simulink model "mw_ssrconverter"  (R2020a)
settings: Solver=VariableStepAuto  StartTime=0.0  StopTime=(8192*2)/256e6  RelTol=1e-3
InitFcn:
  | fs = 256e6;
libraries: hdlsllib x111, simulink x42
(part 1 of 2)
settings Model: EnablePacing=on  PacingRate=0.000001  Creator=david  LastModifiedBy=david
settings OptimizationCC: BlockReduction=off  ConditionallyExecuteInputs=off  DefaultParameterBehavior=Inlined
settings DebuggingCC: AlgebraicLoopMsg=error
settings HardwareCC: ProdBitPerPointer=32  ProdBitPerSizeT=32  ProdBitPerPtrDiffT=32  ProdLargestAtomicFloat=None  ProdIntDivRoundTo=Undefined  ProdEndianess=Unspecified  ProdWordSize=32  ProdHWDeviceType=ASIC/FPGA->ASIC/FPGA  TargetBitPerPointer=64  TargetBitPerSizeT=64  TargetBitPerPtrDiffT=64  TargetLongLongMode=on  TargetIntDivRoundTo=Zero  TargetEndianess=LittleEndian  TargetWordSize=64  TargetHWDeviceType=Custom Processor->MATLAB Host Computer  ProdEqTarget=off

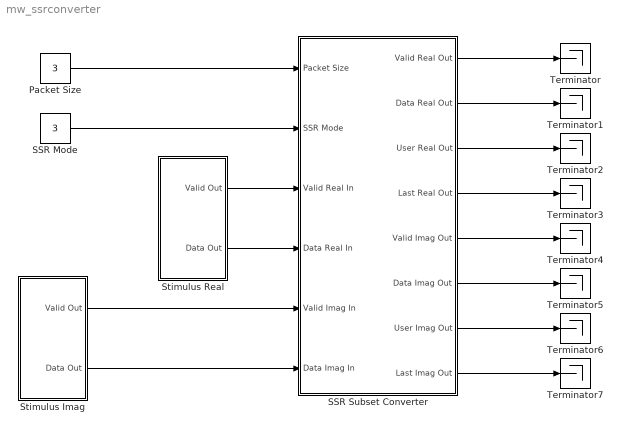
== system mw_ssrconverter ==
  Packet Size : Constant  Value=3  OutDataTypeStr=uint32  SampleTime=-1
  SSR Mode : Constant  Value=3  OutDataTypeStr=uint32  SampleTime=-1
  SSR Subset Converter : Subsystem  TreatAsAtomicUnit=on
  Stimulus Imag : Subsystem
  Stimulus Real : Subsystem
  Terminator{,1..7} (8 alike) : Terminator
  wires:
  Packet Size/1 -> SSR Subset Converter/1(Packet Size)
  SSR Mode/1 -> SSR Subset Converter/2(SSR Mode)
  Stimulus Real/1(Valid Out) -> SSR Subset Converter/3(Valid Real In)
  Stimulus Real/2(Data Out) -> SSR Subset Converter/4(Data Real In)
  SSR Subset Converter/1(Valid Real Out) -> Terminator/1
  SSR Subset Converter/2(Data Real Out) -> Terminator1/1
  SSR Subset Converter/3(User Real Out) -> Terminator2/1
  SSR Subset Converter/4(Last Real Out) -> Terminator3/1
  Stimulus Imag/1(Valid Out) -> SSR Subset Converter/5(Valid Imag In)
  Stimulus Imag/2(Data Out) -> SSR Subset Converter/6(Data Imag In)
  SSR Subset Converter/8(Last Imag Out) -> Terminator7/1
  SSR Subset Converter/7(User Imag Out) -> Terminator6/1
  SSR Subset Converter/6(Data Imag Out) -> Terminator5/1
  SSR Subset Converter/5(Valid Imag Out) -> Terminator4/1

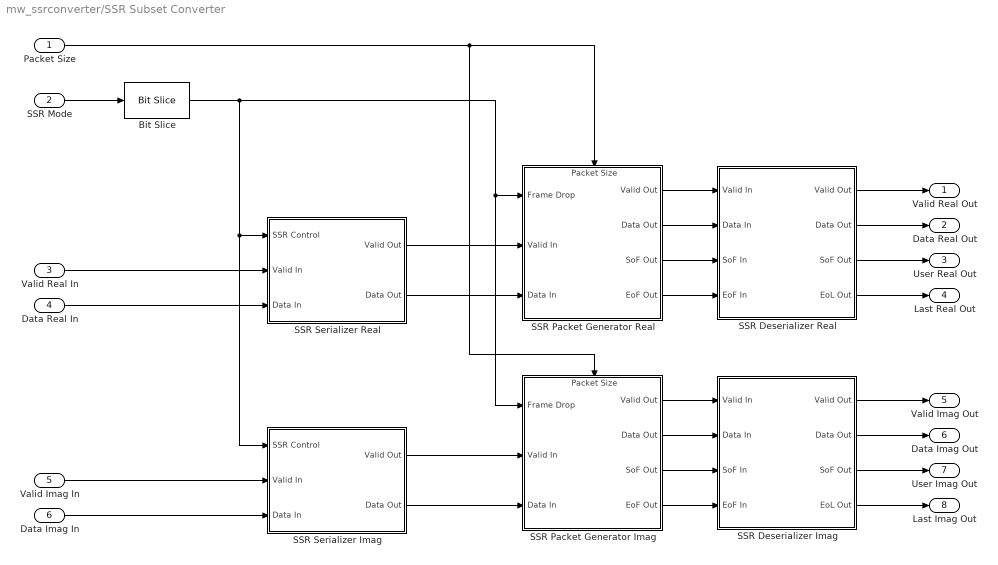
== system mw_ssrconverter/SSR Subset Converter ==
  Packet Size : Inport
  SSR Mode : Inport  Port=2
  Valid Real In : Inport  Port=3
  Data Real In : Inport  Port=4
  Valid Imag In : Inport  Port=5
  Data Imag In : Inport  Port=6
  Bit Slice : hdlsllib/Logic and Bit Operations/Bit Slice  lidx=3  ridx=0
      settings: SourceProductBaseCode=SL
  SSR Deserializer Imag : Subsystem
  SSR Deserializer Real : Subsystem
  SSR Packet Generator Imag : Subsystem
      settings: PortSchema="{\"entries\":[{\"content\":{\"sides\":[{\"content\":{\"connectorIds\":[\"In1\",\"In2\",\"In3\"]},\"type\":\"ConnectorPlacement.EquallySpacedRectSide\",\"uuid\":\"a59bbe9b-b017-421a-b59e-ccf8f0be8c6c\"},{\"content\":{\"connectorIds\":[\"Out1\",\"Out2\",\"Out3\",\"Out4\"],\"side\":\"RIGHT\"},\"type\":\"ConnectorPlacement.EquallySpacedRectSide\",\"uuid\":\"db28a192-666b-40ba-a3e6-dc552d532719\"},{\"content\":{\"connectorIds\":[\"In4\"],\"side\":\"TOP\"},\"type\":\"ConnectorPlacement.EquallySpacedRectSide\",\"uuid\":\"3e188adb-8196-4c2d-ad94-9c10f40ece47\"}]},\"type\":\"ConnectorPlacement.EquallySpacedConnector\",\"uuid\":\"a5800336-434d-4feb-8784-3c17a141dc8c\"}],\"packageUris\":[\"http://schema.mathworks.com/mf0/Connector/19700101\"],\"version\":\"1.0\"}"
  SSR Packet Generator Real : Subsystem
      settings: PortSchema="{\"entries\":[{\"content\":{\"sides\":[{\"content\":{\"connectorIds\":[\"In1\",\"In2\",\"In3\"]},\"type\":\"ConnectorPlacement.EquallySpacedRectSide\",\"uuid\":\"a59bbe9b-b017-421a-b59e-ccf8f0be8c6c\"},{\"content\":{\"connectorIds\":[\"Out1\",\"Out2\",\"Out3\",\"Out4\"],\"side\":\"RIGHT\"},\"type\":\"ConnectorPlacement.EquallySpacedRectSide\",\"uuid\":\"db28a192-666b-40ba-a3e6-dc552d532719\"},{\"content\":{\"connectorIds\":[\"In4\"],\"side\":\"TOP\"},\"type\":\"ConnectorPlacement.EquallySpacedRectSide\",\"uuid\":\"3e188adb-8196-4c2d-ad94-9c10f40ece47\"}]},\"type\":\"ConnectorPlacement.EquallySpacedConnector\",\"uuid\":\"a5800336-434d-4feb-8784-3c17a141dc8c\"}],\"packageUris\":[\"http://schema.mathworks.com/mf0/Connector/19700101\"],\"version\":\"1.0\"}"
  SSR Serializer Imag : Subsystem
  SSR Serializer Real : Subsystem
  Valid Real Out : Outport
  Data Real Out : Outport  Port=2
  User Real Out : Outport  Port=3
  Last Real Out : Outport  Port=4
  Valid Imag Out : Outport  Port=5
  Data Imag Out : Outport  Port=6
  User Imag Out : Outport  Port=7
  Last Imag Out : Outport  Port=8
  wires:
  Data Real In/1 -> SSR Serializer Real/3(Data In)
  SSR Serializer Real/2(Data Out) -> SSR Packet Generator Real/3(Data In)
  SSR Packet Generator Real/4(EoF Out) -> SSR Deserializer Real/4(EoF In)
  SSR Serializer Real/1(Valid Out) -> SSR Packet Generator Real/2(Valid In)
  SSR Deserializer Real/3(SoF Out) -> User Real Out/1
  Bit Slice/1 -> SSR Serializer Imag/1(SSR Control), SSR Serializer Real/1(SSR Control), SSR Packet Generator Imag/1(Frame Drop), SSR Packet Generator Real/1(Frame Drop)
  SSR Packet Generator Real/1(Valid Out) -> SSR Deserializer Real/1(Valid In)
  Valid Real In/1 -> SSR Serializer Real/2(Valid In)
  SSR Packet Generator Real/3(SoF Out) -> SSR Deserializer Real/3(SoF In)
  SSR Packet Generator Real/2(Data Out) -> SSR Deserializer Real/2(Data In)
  SSR Deserializer Real/2(Data Out) -> Data Real Out/1
  SSR Mode/1 -> Bit Slice/1
  SSR Deserializer Real/1(Valid Out) -> Valid Real Out/1
  SSR Deserializer Real/4(EoL Out) -> Last Real Out/1
  Packet Size/1 -> SSR Packet Generator Imag/4(Packet Size), SSR Packet Generator Real/4(Packet Size)
  Valid Imag In/1 -> SSR Serializer Imag/2(Valid In)
  Data Imag In/1 -> SSR Serializer Imag/3(Data In)
  SSR Serializer Imag/1(Valid Out) -> SSR Packet Generator Imag/2(Valid In)
  SSR Serializer Imag/2(Data Out) -> SSR Packet Generator Imag/3(Data In)
  SSR Deserializer Imag/4(EoL Out) -> Last Imag Out/1
  SSR Deserializer Imag/1(Valid Out) -> Valid Imag Out/1
  SSR Deserializer Imag/2(Data Out) -> Data Imag Out/1
  SSR Deserializer Imag/3(SoF Out) -> User Imag Out/1
  SSR Packet Generator Imag/1(Valid Out) -> SSR Deserializer Imag/1(Valid In)
  SSR Packet Generator Imag/2(Data Out) -> SSR Deserializer Imag/2(Data In)
  SSR Packet Generator Imag/3(SoF Out) -> SSR Deserializer Imag/3(SoF In)
  SSR Packet Generator Imag/4(EoF Out) -> SSR Deserializer Imag/4(EoF In)

== system mw_ssrconverter/Stimulus Imag ==
  Constant : Constant  OutDataTypeStr=boolean  SampleTime=1/fs
  Data Type Conversion : DataTypeConversion  OutDataTypeStr=fixdt(0,16,0)
  HDL Counter : hdlsllib/Sources/HDL Counter  CountType=Count limited  CountInit=0  CountStep=8  CountMax=4095  CountFromType=Initial value  CountFrom=0  CountResetPort=off  CountLoadPort=off  CountEnbPort=off  CountDirPort=off  CountDataType=Unsigned  CountWordLen=12  CountFracLen=0  CountSampTime=-1
  HDL Counter1 : hdlsllib/Sources/HDL Counter  CountType=Count limited  CountInit=1  CountStep=8  CountMax=4095  CountFromType=Initial value  CountFrom=1  CountResetPort=off  CountLoadPort=off  CountEnbPort=off  CountDirPort=off  CountDataType=Unsigned  CountWordLen=12  CountFracLen=0  CountSampTime=-1
  HDL Counter2 : hdlsllib/Sources/HDL Counter  CountType=Count limited  CountInit=2  CountStep=8  CountMax=4095  CountFromType=Initial value  CountFrom=2  CountResetPort=off  CountLoadPort=off  CountEnbPort=off  CountDirPort=off  CountDataType=Unsigned  CountWordLen=12  CountFracLen=0  CountSampTime=-1
  HDL Counter3 : hdlsllib/Sources/HDL Counter  CountType=Count limited  CountInit=3  CountStep=8  CountMax=4095  CountFromType=Initial value  CountFrom=3  CountResetPort=off  CountLoadPort=off  CountEnbPort=off  CountDirPort=off  CountDataType=Unsigned  CountWordLen=12  CountFracLen=0  CountSampTime=-1
  HDL Counter4 : hdlsllib/Sources/HDL Counter  CountType=Count limited  CountInit=4  CountStep=8  CountMax=4095  CountFromType=Initial value  CountFrom=4  CountResetPort=off  CountLoadPort=off  CountEnbPort=off  CountDirPort=off  CountDataType=Unsigned  CountWordLen=12  CountFracLen=0  CountSampTime=-1
  HDL Counter5 : hdlsllib/Sources/HDL Counter  CountType=Count limited  CountInit=5  CountStep=8  CountMax=4095  CountFromType=Initial value  CountFrom=5  CountResetPort=off  CountLoadPort=off  CountEnbPort=off  CountDirPort=off  CountDataType=Unsigned  CountWordLen=12  CountFracLen=0  CountSampTime=-1
  HDL Counter6 : hdlsllib/Sources/HDL Counter  CountType=Count limited  CountInit=6  CountStep=8  CountMax=4095  CountFromType=Initial value  CountFrom=6  CountResetPort=off  CountLoadPort=off  CountEnbPort=off  CountDirPort=off  CountDataType=Unsigned  CountWordLen=12  CountFracLen=0  CountSampTime=-1
  HDL Counter7 : hdlsllib/Sources/HDL Counter  CountType=Count limited  CountInit=7  CountStep=8  CountMax=4095  CountFromType=Initial value  CountFrom=7  CountResetPort=off  CountLoadPort=off  CountEnbPort=off  CountDirPort=off  CountDataType=Unsigned  CountWordLen=12  CountFracLen=0  CountSampTime=-1
  Vector Concatenate : Concatenate  NumInputs=8
  Vector to SSR : Subsystem  mask{N=8, hN=8}
      mask prompts: N "Samples per clock cycle:"
      mask init:
      | if ~isequal(get_param(gcb, 'N'), get_param(gcb, 'hN'))
      |     % Delete all blocks except input and output ports
      |     delete_block(setxor(setdiff(...
      |         find_system(gcb,'LookUnderMasks','on'),...
      |         {[gcb, '/Vector'], [gcb, '/SSR']}), gcb));
      | 
      |     % Delete all wires
      |     delete_line(find_system(gcb, 'FindAll', 'on', 'LookUnderMasks',...
      |         'on', 'SearchDepth', 3, 'Type', 'line', 'Connected', 'off'));
      | 
      |     % Add the bit concatenation block
      |     add_block('hdlsllib/Logic and Bit Operations/Bit Concat',...
      |         [gcb, '/Bit Concat'],...
      |         'Position', [155 55 205 330]);
      |     set_param([gcb, '/Bit Concat'], 'numInputs', num2str(N));
      | 
      |     % Add wire to output
      |     add_line(gcb, 'Bit Concat/1', 'SSR/1');
      | 
      |     % Add selector blocks and connect wires
      |     for i = 0:N-1
      |         add_block('simulink/Signal Routing/Selector',...
      |             [gcb, '/Selector', num2str(i)],...
      |             'Position', [0 82+i*90 45 128+i*90]);
      |         set_param([gcb, '/Selector', num2str(i)], 'InputPortWidth', num2str(N));
      |         set_param([gcb, '/Selector', num2str(i)], 'IndexParamArray', {num2str(N-i)});
      |         add_line(gcb, 'Vector/1', ['Selector', num2str(i), '/1'],...
      |             'autorouting', 'on');
      |         add_line(gcb, ['Selector', num2str(i), '/1'],...
      |             ['Bit Concat/', num2str(i+1)],...
      |             'autorouting', 'on');
      |     end
      |     
      |     % Set the hidden attribute to prevent unnecessary changes in
      |     % architecture while generating HDL Code.
      |     set_param(gcb, 'hN', get_param(gcb, 'N'));
      | end
      mask DialogControl DescGroupVar Prompt: Vector to SSR
      mask DialogControl DescTextVar Prompt: Convert a vector of inputs into SSR format.
  Valid Out : Outport
  Data Out : Outport  Port=2
  wires:
  Vector to SSR/1(SSR) -> Data Out/1
  Data Type Conversion/1 -> Vector to SSR/1(Vector)
  HDL Counter/1 -> Vector Concatenate/1
  HDL Counter1/1 -> Vector Concatenate/2
  HDL Counter2/1 -> Vector Concatenate/3
  HDL Counter3/1 -> Vector Concatenate/4
  HDL Counter4/1 -> Vector Concatenate/5
  HDL Counter5/1 -> Vector Concatenate/6
  HDL Counter6/1 -> Vector Concatenate/7
  HDL Counter7/1 -> Vector Concatenate/8
  Constant/1 -> Valid Out/1
  Vector Concatenate/1 -> Data Type Conversion/1

== system mw_ssrconverter/Stimulus Real ==
  Constant : Constant  OutDataTypeStr=boolean  SampleTime=1/fs
  Data Type Conversion : DataTypeConversion  OutDataTypeStr=fixdt(0,16,0)
  HDL Counter : hdlsllib/Sources/HDL Counter  CountType=Count limited  CountInit=0  CountStep=8  CountMax=4095  CountFromType=Initial value  CountFrom=0  CountResetPort=off  CountLoadPort=off  CountEnbPort=off  CountDirPort=off  CountDataType=Unsigned  CountWordLen=12  CountFracLen=0  CountSampTime=-1
  HDL Counter1 : hdlsllib/Sources/HDL Counter  CountType=Count limited  CountInit=1  CountStep=8  CountMax=4095  CountFromType=Initial value  CountFrom=1  CountResetPort=off  CountLoadPort=off  CountEnbPort=off  CountDirPort=off  CountDataType=Unsigned  CountWordLen=12  CountFracLen=0  CountSampTime=-1
  HDL Counter2 : hdlsllib/Sources/HDL Counter  CountType=Count limited  CountInit=2  CountStep=8  CountMax=4095  CountFromType=Initial value  CountFrom=2  CountResetPort=off  CountLoadPort=off  CountEnbPort=off  CountDirPort=off  CountDataType=Unsigned  CountWordLen=12  CountFracLen=0  CountSampTime=-1
  HDL Counter3 : hdlsllib/Sources/HDL Counter  CountType=Count limited  CountInit=3  CountStep=8  CountMax=4095  CountFromType=Initial value  CountFrom=3  CountResetPort=off  CountLoadPort=off  CountEnbPort=off  CountDirPort=off  CountDataType=Unsigned  CountWordLen=12  CountFracLen=0  CountSampTime=-1
  HDL Counter4 : hdlsllib/Sources/HDL Counter  CountType=Count limited  CountInit=4  CountStep=8  CountMax=4095  CountFromType=Initial value  CountFrom=4  CountResetPort=off  CountLoadPort=off  CountEnbPort=off  CountDirPort=off  CountDataType=Unsigned  CountWordLen=12  CountFracLen=0  CountSampTime=-1
  HDL Counter5 : hdlsllib/Sources/HDL Counter  CountType=Count limited  CountInit=5  CountStep=8  CountMax=4095  CountFromType=Initial value  CountFrom=5  CountResetPort=off  CountLoadPort=off  CountEnbPort=off  CountDirPort=off  CountDataType=Unsigned  CountWordLen=12  CountFracLen=0  CountSampTime=-1
  HDL Counter6 : hdlsllib/Sources/HDL Counter  CountType=Count limited  CountInit=6  CountStep=8  CountMax=4095  CountFromType=Initial value  CountFrom=6  CountResetPort=off  CountLoadPort=off  CountEnbPort=off  CountDirPort=off  CountDataType=Unsigned  CountWordLen=12  CountFracLen=0  CountSampTime=-1
  HDL Counter7 : hdlsllib/Sources/HDL Counter  CountType=Count limited  CountInit=7  CountStep=8  CountMax=4095  CountFromType=Initial value  CountFrom=7  CountResetPort=off  CountLoadPort=off  CountEnbPort=off  CountDirPort=off  CountDataType=Unsigned  CountWordLen=12  CountFracLen=0  CountSampTime=-1
  Vector Concatenate : Concatenate  NumInputs=8
  Vector to SSR : Subsystem  mask{N=8, hN=8}
      mask prompts: N "Samples per clock cycle:"
      mask init: same as mw_ssrconverter/Stimulus Imag/Vector to SSR
      mask DialogControl DescGroupVar Prompt: Vector to SSR
      mask DialogControl DescTextVar Prompt: Convert a vector of inputs into SSR format.
  Valid Out : Outport
  Data Out : Outport  Port=2
  wires:
  Vector Concatenate/1 -> Data Type Conversion/1
  Constant/1 -> Valid Out/1
  HDL Counter7/1 -> Vector Concatenate/8
  HDL Counter6/1 -> Vector Concatenate/7
  HDL Counter5/1 -> Vector Concatenate/6
  HDL Counter4/1 -> Vector Concatenate/5
  HDL Counter3/1 -> Vector Concatenate/4
  HDL Counter2/1 -> Vector Concatenate/3
  HDL Counter1/1 -> Vector Concatenate/2
  HDL Counter/1 -> Vector Concatenate/1
  Data Type Conversion/1 -> Vector to SSR/1(Vector)
  Vector to SSR/1(SSR) -> Data Out/1

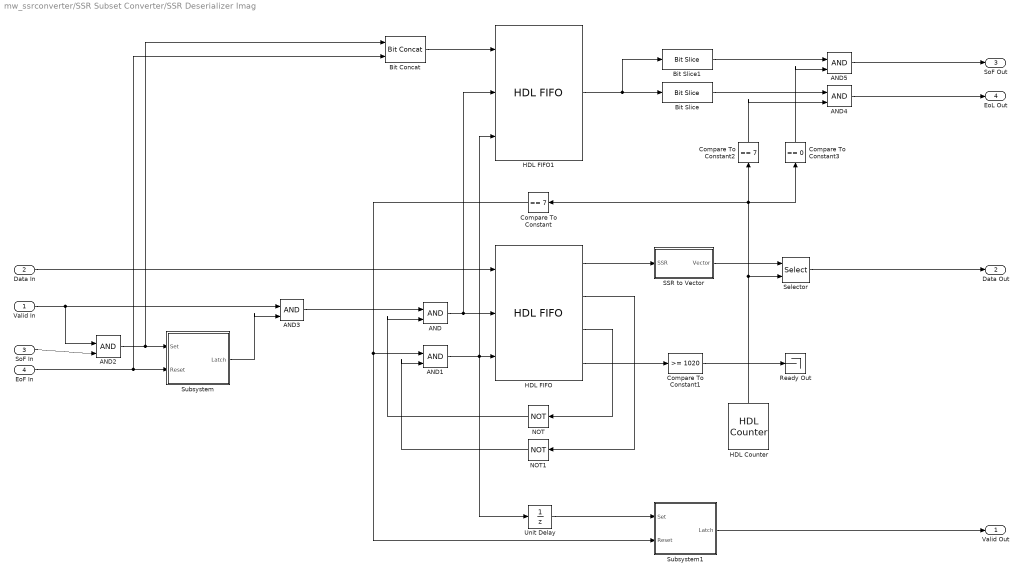
== system mw_ssrconverter/SSR Subset Converter/SSR Deserializer Imag ==
  Valid In : Inport
  Data In : Inport  Port=2
  SoF In : Inport  Port=3
  EoF In : Inport  Port=4
  AND{,1..5} (6 alike) : Logic  IconShape=distinctive  AllPortsSameDT=off  OutDataTypeStr=boolean
  Bit Concat : hdlsllib/Logic and Bit Operations/Bit Concat  numInputs=2
  Bit Slice : hdlsllib/Logic and Bit Operations/Bit Slice  lidx=0  ridx=0
      settings: SourceProductBaseCode=SL
  Bit Slice1 : hdlsllib/Logic and Bit Operations/Bit Slice  lidx=1  ridx=1
      settings: SourceProductBaseCode=SL
  Compare To Constant : simulink/Logic and Bit Operations/Compare To Constant  relop===  const=7  OutDataTypeStr=boolean
  Compare To Constant1 : simulink/Logic and Bit Operations/Compare To Constant  relop=>=  const=1020  OutDataTypeStr=boolean
  Compare To Constant2 : simulink/Logic and Bit Operations/Compare To Constant  relop===  const=7  OutDataTypeStr=boolean
  Compare To Constant3 : simulink/Logic and Bit Operations/Compare To Constant  relop===  const=0  OutDataTypeStr=boolean
  HDL Counter : hdlsllib/Sources/HDL Counter  CountType=Count limited  CountInit=0  CountStep=1  CountMax=7  CountFromType=Initial value  CountFrom=0  CountResetPort=off  CountLoadPort=off  CountEnbPort=off  CountDirPort=off  CountDataType=Unsigned  CountWordLen=8  CountFracLen=0  CountSampTime=-1
  HDL FIFO : hdlsllib/HDL RAMs/HDL FIFO  fifo_size=1024  mode=Classic  ratio=1  push_msg=Error  pop_msg=Error  show_empty=on  show_full=on  show_num=on  LabelModeActiveChoice_Mode=Classic
      settings: SourceProductBaseCode=SL
  HDL FIFO1 : hdlsllib/HDL RAMs/HDL FIFO  fifo_size=1024  mode=Classic  ratio=1  push_msg=Error  pop_msg=Error  show_empty=off  show_full=off  show_num=off  LabelModeActiveChoice_Mode=Classic
      settings: SourceProductBaseCode=SL
  NOT : Logic  Operator=NOT  IconShape=distinctive  AllPortsSameDT=off  OutDataTypeStr=boolean
  NOT1 : Logic  Operator=NOT  IconShape=distinctive  AllPortsSameDT=off  OutDataTypeStr=boolean
  Ready Out : Terminator
  SSR to Vector : Subsystem  mask{N=8, w=16, hN=8, hw=16}
      mask prompts: N "Samples per clock cycle:"; w "Wordlength:"
      mask init:
      | if ~isequal(get_param(gcb, 'N'), get_param(gcb, 'hN')) ||...
      |         ~isequal(get_param(gcb, 'w'), get_param(gcb, 'hw'))
      |     % Delete all blocks except input and output ports
      |     delete_block(setxor(setdiff(...
      |         find_system(gcb,'LookUnderMasks','on'),...
      |         {[gcb, '/Vector'], [gcb, '/SSR']}), gcb));
      | 
      |     % Delete all wires
      |     delete_line(find_system(gcb, 'FindAll', 'on', 'LookUnderMasks',...
      |         'on', 'SearchDepth', 3, 'Type', 'line', 'Connected', 'off'));
      | 
      |     % Add the matrix concatenation block
      |     add_block('hdlsllib/Math Operations/Matrix Concatenate',...
      |         [gcb, '/Matrix Concatenate'],...
      |         'Position', [155 55 205 330]);
      |     set_param([gcb, '/Matrix Concatenate'], 'NumInputs', num2str(N));
      |     set_param([gcb, '/Matrix Concatenate'], 'Mode', 'Vector');
      |     
      |     % Add wire to output
      |     add_line(gcb, 'Matrix Concatenate/1', 'Vector/1');
      | 
      |     % Add slice blocks and connect wires
      |     for i = 0:N-1
      |         add_block('hdlsllib/Logic and Bit Operations/Bit Slice',...
      |             [gcb, '/Bit Slice', num2str(i)],...
      |             'Position', [0 82+i*90 45 128+i*90]);
      |         set_param([gcb, '/Bit Slice', num2str(i)], 'ridx', num2str(0+i*(w)));
      |         set_param([gcb, '/Bit Slice', num2str(i)], 'lidx', num2str((w-1)+i*(w)));
      |         add_line(gcb, 'SSR/1', ['Bit Slice', num2str(i), '/1'],...
      |             'autorouting', 'on');
      |         add_line(gcb, ['Bit Slice', num2str(i), '/1'],...
      |             ['Matrix Concatenate/', num2str(i+1)],...
      |             'autorouting', 'on');
      |     end
      |     
      |     % Set the hidden attribute to prevent unnecessary changes in
      |     % architecture while generating HDL Code.
      |     set_param(gcb, 'hN', get_param(gcb, 'N'));
      |     set_param(gcb, 'hw', get_param(gcb, 'w'));
      | end
      mask DialogControl DescGroupVar Prompt: SSR to Vector
      mask DialogControl DescTextVar Prompt: Convert the SSR vector format based on the wordlength and expected number of samples per clock cycle.
  Selector : Selector  IndexMode=Zero-based  InputPortWidth=8  IndexOptions=Index vector (port)  Indices=[1 3]  OutputSizes=1
  Subsystem : Subsystem
  Subsystem1 : Subsystem
  Unit Delay : UnitDelay  SampleTime=-1  HasFrameUpgradeWarning=on
  Valid Out : Outport
  Data Out : Outport  Port=2
  SoF Out : Outport  Port=3
  EoL Out : Outport  Port=4
  wires:
  Selector/1 -> Data Out/1
  SSR to Vector/1(Vector) -> Selector/1
  Data In/1 -> HDL FIFO/1
  Compare To Constant1/1 -> Ready Out/1
  AND5/1 -> SoF Out/1
  AND4/1 -> EoL Out/1
  Compare To Constant3/1 -> AND5/2
  Bit Slice1/1 -> AND5/1
  Bit Slice/1 -> AND4/1
  Compare To Constant2/1 -> AND4/2
  HDL FIFO1/1 -> Bit Slice/1, Bit Slice1/1
  Bit Concat/1 -> HDL FIFO1/1
  Subsystem/1(Latch) -> AND3/2
  HDL FIFO/4 -> Compare To Constant1/1
  Subsystem1/1(Latch) -> Valid Out/1
  NOT1/1 -> AND1/2
  HDL FIFO/2 -> NOT1/1
  Unit Delay/1 -> Subsystem1/1(Set)
  NOT/1 -> AND/2
  EoF In/1 -> Subsystem/2(Reset), Bit Concat/2
  AND3/1 -> AND/1
  Compare To Constant/1 -> AND1/1, Subsystem1/2(Reset)
  AND2/1 -> Subsystem/1(Set), Bit Concat/1
  Valid In/1 -> AND2/1, AND3/1
  SoF In/1 -> AND2/2
  HDL FIFO/3 -> NOT/1
  AND1/1 -> HDL FIFO/3, HDL FIFO1/3, Unit Delay/1
  AND/1 -> HDL FIFO1/2, HDL FIFO/2
  HDL Counter/1 -> Selector/2, Compare To Constant/1, Compare To Constant2/1, Compare To Constant3/1
  HDL FIFO/1 -> SSR to Vector/1(SSR)

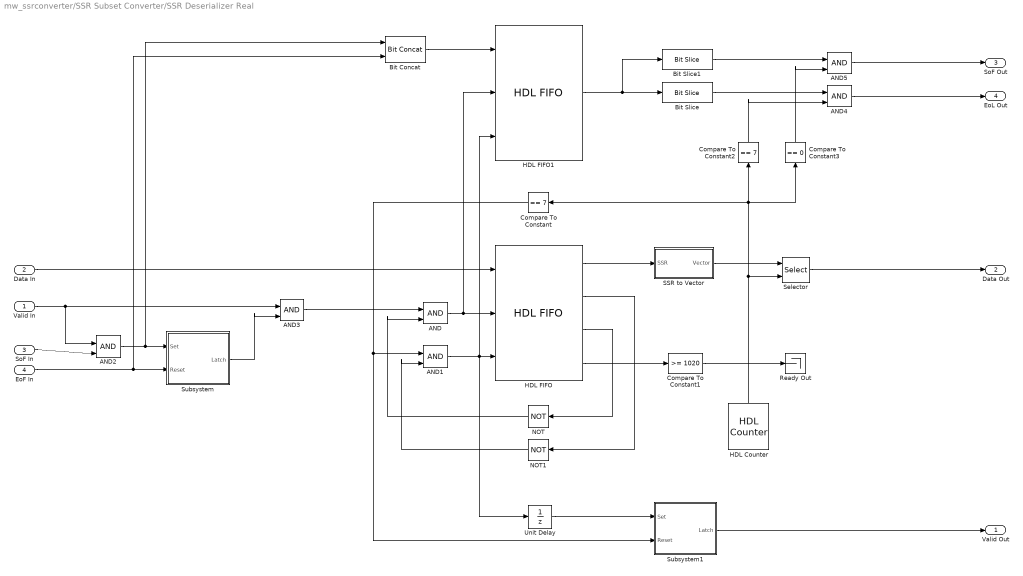
== system mw_ssrconverter/SSR Subset Converter/SSR Deserializer Real ==
  Valid In : Inport
  Data In : Inport  Port=2
  SoF In : Inport  Port=3
  EoF In : Inport  Port=4
  AND{,1..5} (6 alike) : Logic  IconShape=distinctive  AllPortsSameDT=off  OutDataTypeStr=boolean
  Bit Concat : hdlsllib/Logic and Bit Operations/Bit Concat  numInputs=2
  Bit Slice : hdlsllib/Logic and Bit Operations/Bit Slice  lidx=0  ridx=0
      settings: SourceProductBaseCode=SL
  Bit Slice1 : hdlsllib/Logic and Bit Operations/Bit Slice  lidx=1  ridx=1
      settings: SourceProductBaseCode=SL
  Compare To Constant : simulink/Logic and Bit Operations/Compare To Constant  relop===  const=7  OutDataTypeStr=boolean
  Compare To Constant1 : simulink/Logic and Bit Operations/Compare To Constant  relop=>=  const=1020  OutDataTypeStr=boolean
  Compare To Constant2 : simulink/Logic and Bit Operations/Compare To Constant  relop===  const=7  OutDataTypeStr=boolean
  Compare To Constant3 : simulink/Logic and Bit Operations/Compare To Constant  relop===  const=0  OutDataTypeStr=boolean
  HDL Counter : hdlsllib/Sources/HDL Counter  CountType=Count limited  CountInit=0  CountStep=1  CountMax=7  CountFromType=Initial value  CountFrom=0  CountResetPort=off  CountLoadPort=off  CountEnbPort=off  CountDirPort=off  CountDataType=Unsigned  CountWordLen=8  CountFracLen=0  CountSampTime=-1
  HDL FIFO : hdlsllib/HDL RAMs/HDL FIFO  fifo_size=1024  mode=Classic  ratio=1  push_msg=Error  pop_msg=Error  show_empty=on  show_full=on  show_num=on  LabelModeActiveChoice_Mode=Classic
      settings: SourceProductBaseCode=SL
  HDL FIFO1 : hdlsllib/HDL RAMs/HDL FIFO  fifo_size=1024  mode=Classic  ratio=1  push_msg=Error  pop_msg=Error  show_empty=off  show_full=off  show_num=off  LabelModeActiveChoice_Mode=Classic
      settings: SourceProductBaseCode=SL
  NOT : Logic  Operator=NOT  IconShape=distinctive  AllPortsSameDT=off  OutDataTypeStr=boolean
  NOT1 : Logic  Operator=NOT  IconShape=distinctive  AllPortsSameDT=off  OutDataTypeStr=boolean
  Ready Out : Terminator
  SSR to Vector : Subsystem  mask{N=8, w=16, hN=8, hw=16}
      mask prompts: N "Samples per clock cycle:"; w "Wordlength:"
      mask init: same as mw_ssrconverter/SSR Subset Converter/SSR Deserializer Imag/SSR to Vector
      mask DialogControl DescGroupVar Prompt: SSR to Vector
      mask DialogControl DescTextVar Prompt: Convert the SSR vector format based on the wordlength and expected number of samples per clock cycle.
  Selector : Selector  IndexMode=Zero-based  InputPortWidth=8  IndexOptions=Index vector (port)  Indices=[1 3]  OutputSizes=1
  Subsystem : Subsystem
  Subsystem1 : Subsystem
  Unit Delay : UnitDelay  SampleTime=-1  HasFrameUpgradeWarning=on
  Valid Out : Outport
  Data Out : Outport  Port=2
  SoF Out : Outport  Port=3
  EoL Out : Outport  Port=4
  wires:
  HDL FIFO/1 -> SSR to Vector/1(SSR)
  HDL Counter/1 -> Compare To Constant3/1, Compare To Constant2/1, Compare To Constant/1, Selector/2
  AND/1 -> HDL FIFO/2, HDL FIFO1/2
  AND1/1 -> Unit Delay/1, HDL FIFO1/3, HDL FIFO/3
  HDL FIFO/3 -> NOT/1
  SoF In/1 -> AND2/2
  Valid In/1 -> AND3/1, AND2/1
  AND2/1 -> Bit Concat/1, Subsystem/1(Set)
  Compare To Constant/1 -> Subsystem1/2(Reset), AND1/1
  AND3/1 -> AND/1
  EoF In/1 -> Bit Concat/2, Subsystem/2(Reset)
  NOT/1 -> AND/2
  Unit Delay/1 -> Subsystem1/1(Set)
  HDL FIFO/2 -> NOT1/1
  NOT1/1 -> AND1/2
  Subsystem1/1(Latch) -> Valid Out/1
  HDL FIFO/4 -> Compare To Constant1/1
  Subsystem/1(Latch) -> AND3/2
  Bit Concat/1 -> HDL FIFO1/1
  HDL FIFO1/1 -> Bit Slice1/1, Bit Slice/1
  Compare To Constant2/1 -> AND4/2
  Bit Slice/1 -> AND4/1
  Bit Slice1/1 -> AND5/1
  Compare To Constant3/1 -> AND5/2
  AND4/1 -> EoL Out/1
  AND5/1 -> SoF Out/1
  Compare To Constant1/1 -> Ready Out/1
  Data In/1 -> HDL FIFO/1
  SSR to Vector/1(Vector) -> Selector/1
  Selector/1 -> Data Out/1

== system mw_ssrconverter/SSR Subset Converter/SSR Packet Generator Imag ==
  Frame Drop : Inport
  Valid In : Inport  Port=2
  Data In : Inport  Port=3
  Packet Size : Inport  Port=4
  Frame Dropper : Subsystem
      settings: PortSchema="{\"entries\":[{\"content\":{\"sides\":[{\"content\":{\"connectorIds\":[\"In1\",\"In2\",\"In3\",\"In4\"]},\"type\":\"ConnectorPlacement.EquallySpacedRectSide\",\"uuid\":\"54c30b66-c84f-403b-ae2b-65cc6aec53ae\"},{\"content\":{\"connectorIds\":[\"Out1\",\"Out2\",\"Out3\",\"Out4\"],\"side\":\"RIGHT\"},\"type\":\"ConnectorPlacement.EquallySpacedRectSide\",\"uuid\":\"7fa28ff6-8fce-4ceb-b755-50de3dfb11ba\"},{\"content\":{\"connectorIds\":[\"In5\"],\"side\":\"TOP\"},\"type\":\"ConnectorPlacement.EquallySpacedRectSide\",\"uuid\":\"f3e3849e-6de4-4089-b190-2f6ddd7da8c2\"}]},\"type\":\"ConnectorPlacement.EquallySpacedConnector\",\"uuid\":\"90f0c780-b61a-4293-8926-b92d09c8458c\"}],\"packageUris\":[\"http://schema.mathworks.com/mf0/Connector/19700101\"],\"version\":\"1.0\"}"
  TLAST Generator : Subsystem
  Valid Out : Outport
  Data Out : Outport  Port=2
  SoF Out : Outport  Port=3
  EoF Out : Outport  Port=4
  wires:
  Frame Drop/1 -> Frame Dropper/5(Frame Drop)
  TLAST Generator/4(EoF Out) -> Frame Dropper/4(EoF In)
  TLAST Generator/3(SoF Out) -> Frame Dropper/3(SoF In)
  Frame Dropper/1(Valid Out) -> Valid Out/1
  Frame Dropper/2(Data Out) -> Data Out/1
  Frame Dropper/4(EoF Out) -> EoF Out/1
  Frame Dropper/3(SoF Out) -> SoF Out/1
  TLAST Generator/2(Data Out) -> Frame Dropper/2(Data In)
  TLAST Generator/1(Valid Out) -> Frame Dropper/1(Valid In)
  Packet Size/1 -> TLAST Generator/3(Packet Size)
  Data In/1 -> TLAST Generator/2(Data In)
  Valid In/1 -> TLAST Generator/1(Valid In)

== system mw_ssrconverter/SSR Subset Converter/SSR Packet Generator Real ==
  Frame Drop : Inport
  Valid In : Inport  Port=2
  Data In : Inport  Port=3
  Packet Size : Inport  Port=4
  Frame Dropper : Subsystem
      settings: PortSchema="{\"entries\":[{\"content\":{\"sides\":[{\"content\":{\"connectorIds\":[\"In1\",\"In2\",\"In3\",\"In4\"]},\"type\":\"ConnectorPlacement.EquallySpacedRectSide\",\"uuid\":\"54c30b66-c84f-403b-ae2b-65cc6aec53ae\"},{\"content\":{\"connectorIds\":[\"Out1\",\"Out2\",\"Out3\",\"Out4\"],\"side\":\"RIGHT\"},\"type\":\"ConnectorPlacement.EquallySpacedRectSide\",\"uuid\":\"7fa28ff6-8fce-4ceb-b755-50de3dfb11ba\"},{\"content\":{\"connectorIds\":[\"In5\"],\"side\":\"TOP\"},\"type\":\"ConnectorPlacement.EquallySpacedRectSide\",\"uuid\":\"f3e3849e-6de4-4089-b190-2f6ddd7da8c2\"}]},\"type\":\"ConnectorPlacement.EquallySpacedConnector\",\"uuid\":\"90f0c780-b61a-4293-8926-b92d09c8458c\"}],\"packageUris\":[\"http://schema.mathworks.com/mf0/Connector/19700101\"],\"version\":\"1.0\"}"
  TLAST Generator : Subsystem
  Valid Out : Outport
  Data Out : Outport  Port=2
  SoF Out : Outport  Port=3
  EoF Out : Outport  Port=4
  wires:
  Valid In/1 -> TLAST Generator/1(Valid In)
  Data In/1 -> TLAST Generator/2(Data In)
  Packet Size/1 -> TLAST Generator/3(Packet Size)
  TLAST Generator/1(Valid Out) -> Frame Dropper/1(Valid In)
  TLAST Generator/2(Data Out) -> Frame Dropper/2(Data In)
  Frame Dropper/3(SoF Out) -> SoF Out/1
  Frame Dropper/4(EoF Out) -> EoF Out/1
  Frame Dropper/2(Data Out) -> Data Out/1
  Frame Dropper/1(Valid Out) -> Valid Out/1
  TLAST Generator/3(SoF Out) -> Frame Dropper/3(SoF In)
  TLAST Generator/4(EoF Out) -> Frame Dropper/4(EoF In)
  Frame Drop/1 -> Frame Dropper/5(Frame Drop)

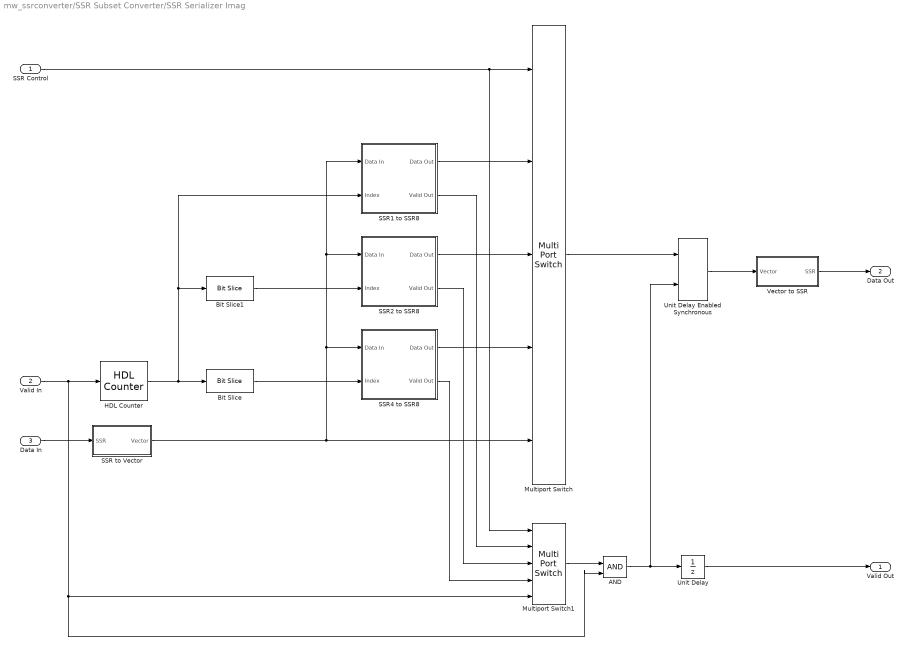
== system mw_ssrconverter/SSR Subset Converter/SSR Serializer Imag ==
  SSR Control : Inport
  Valid In : Inport  Port=2
  Data In : Inport  Port=3
  AND : Logic  IconShape=distinctive  AllPortsSameDT=off  OutDataTypeStr=boolean
  Bit Slice : hdlsllib/Logic and Bit Operations/Bit Slice  lidx=0  ridx=0
      settings: SourceProductBaseCode=SL
  Bit Slice1 : hdlsllib/Logic and Bit Operations/Bit Slice  lidx=1  ridx=0
      settings: SourceProductBaseCode=SL
  HDL Counter : hdlsllib/Sources/HDL Counter  CountType=Count limited  CountInit=0  CountStep=1  CountMax=7  CountFromType=Initial value  CountFrom=0  CountResetPort=off  CountLoadPort=off  CountEnbPort=on  CountDirPort=off  CountDataType=Unsigned  CountWordLen=3  CountFracLen=0  CountSampTime=1
  Multiport Switch : MultiPortSwitch  DataPortOrder=Zero-based contiguous  Inputs=4  zeroidx=on
  Multiport Switch1 : MultiPortSwitch  DataPortOrder=Zero-based contiguous  Inputs=4  zeroidx=on
  SSR to Vector : Subsystem  mask{N=8, w=16, hN=8, hw=16}
      mask prompts: N "Samples per clock cycle:"; w "Wordlength:"
      mask init: same as mw_ssrconverter/SSR Subset Converter/SSR Deserializer Imag/SSR to Vector
      mask DialogControl DescGroupVar Prompt: SSR to Vector
      mask DialogControl DescTextVar Prompt: Convert the SSR vector format based on the wordlength and expected number of samples per clock cycle.
  SSR1 to SSR8 : Subsystem
  SSR2 to SSR8 : Subsystem
  SSR4 to SSR8 : Subsystem
  Unit Delay : UnitDelay  SampleTime=-1  HasFrameUpgradeWarning=on
  Unit Delay Enabled Synchronous : hdlsllib/Discrete/Unit Delay Enabled Synchronous  InitialCondition=0.0  SampleTime=-1
      settings: SourceProductBaseCode=SL
  Vector to SSR : Subsystem  mask{N=8, hN=8}
      mask prompts: N "Samples per clock cycle:"
      mask init: same as mw_ssrconverter/Stimulus Imag/Vector to SSR
      mask DialogControl DescGroupVar Prompt: Vector to SSR
      mask DialogControl DescTextVar Prompt: Convert a vector of inputs into SSR format.
  Valid Out : Outport
  Data Out : Outport  Port=2
  wires:
  Vector to SSR/1(SSR) -> Data Out/1
  SSR to Vector/1(Vector) -> SSR4 to SSR8/1(Data In), SSR2 to SSR8/1(Data In), SSR1 to SSR8/1(Data In), Multiport Switch/5
  Unit Delay Enabled Synchronous/1 -> Vector to SSR/1(Vector)
  Multiport Switch/1 -> Unit Delay Enabled Synchronous/1
  Unit Delay/1 -> Valid Out/1
  Valid In/1 -> HDL Counter/1, Multiport Switch1/5, AND/2
  AND/1 -> Unit Delay/1, Unit Delay Enabled Synchronous/2
  Multiport Switch1/1 -> AND/1
  SSR4 to SSR8/2(Valid Out) -> Multiport Switch1/4
  SSR2 to SSR8/2(Valid Out) -> Multiport Switch1/3
  SSR1 to SSR8/2(Valid Out) -> Multiport Switch1/2
  Bit Slice/1 -> SSR4 to SSR8/2(Index)
  SSR Control/1 -> Multiport Switch/1, Multiport Switch1/1
  HDL Counter/1 -> SSR1 to SSR8/2(Index), Bit Slice1/1, Bit Slice/1
  Bit Slice1/1 -> SSR2 to SSR8/2(Index)
  Data In/1 -> SSR to Vector/1(SSR)
  SSR1 to SSR8/1(Data Out) -> Multiport Switch/2
  SSR2 to SSR8/1(Data Out) -> Multiport Switch/3
  SSR4 to SSR8/1(Data Out) -> Multiport Switch/4

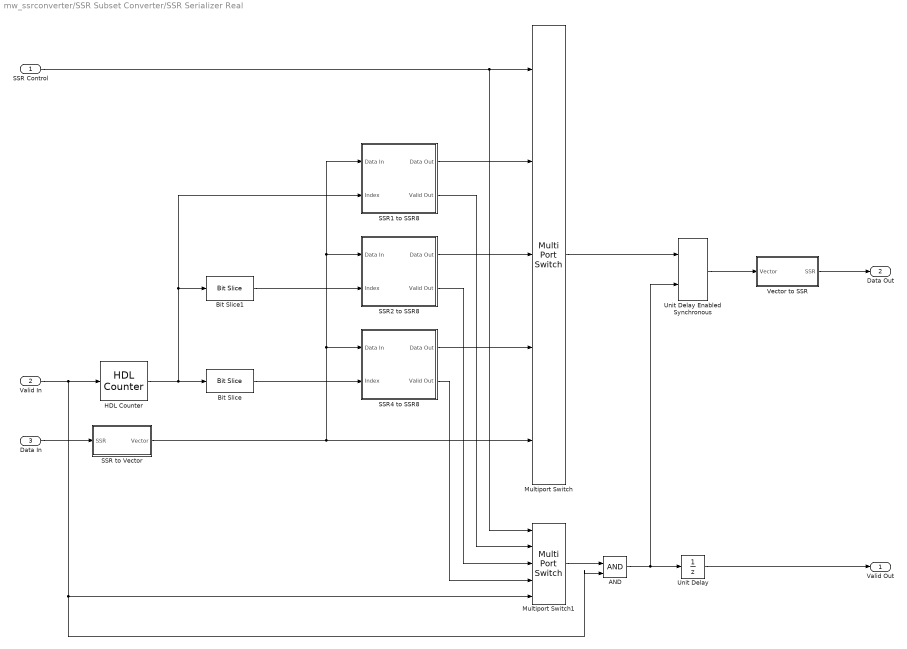
== system mw_ssrconverter/SSR Subset Converter/SSR Serializer Real ==
  SSR Control : Inport
  Valid In : Inport  Port=2
  Data In : Inport  Port=3
  AND : Logic  IconShape=distinctive  AllPortsSameDT=off  OutDataTypeStr=boolean
  Bit Slice : hdlsllib/Logic and Bit Operations/Bit Slice  lidx=0  ridx=0
      settings: SourceProductBaseCode=SL
  Bit Slice1 : hdlsllib/Logic and Bit Operations/Bit Slice  lidx=1  ridx=0
      settings: SourceProductBaseCode=SL
  HDL Counter : hdlsllib/Sources/HDL Counter  CountType=Count limited  CountInit=0  CountStep=1  CountMax=7  CountFromType=Initial value  CountFrom=0  CountResetPort=off  CountLoadPort=off  CountEnbPort=on  CountDirPort=off  CountDataType=Unsigned  CountWordLen=3  CountFracLen=0  CountSampTime=1
  Multiport Switch : MultiPortSwitch  DataPortOrder=Zero-based contiguous  Inputs=4  zeroidx=on
  Multiport Switch1 : MultiPortSwitch  DataPortOrder=Zero-based contiguous  Inputs=4  zeroidx=on
  SSR to Vector : Subsystem  mask{N=8, w=16, hN=8, hw=16}
      mask prompts: N "Samples per clock cycle:"; w "Wordlength:"
      mask init: same as mw_ssrconverter/SSR Subset Converter/SSR Deserializer Imag/SSR to Vector
      mask DialogControl DescGroupVar Prompt: SSR to Vector
      mask DialogControl DescTextVar Prompt: Convert the SSR vector format based on the wordlength and expected number of samples per clock cycle.
  SSR1 to SSR8 : Subsystem
  SSR2 to SSR8 : Subsystem
  SSR4 to SSR8 : Subsystem
  Unit Delay : UnitDelay  SampleTime=-1  HasFrameUpgradeWarning=on
  Unit Delay Enabled Synchronous : hdlsllib/Discrete/Unit Delay Enabled Synchronous  InitialCondition=0.0  SampleTime=-1
      settings: SourceProductBaseCode=SL
  Vector to SSR : Subsystem  mask{N=8, hN=8}
      mask prompts: N "Samples per clock cycle:"
      mask init: same as mw_ssrconverter/Stimulus Imag/Vector to SSR
      mask DialogControl DescGroupVar Prompt: Vector to SSR
      mask DialogControl DescTextVar Prompt: Convert a vector of inputs into SSR format.
  Valid Out : Outport
  Data Out : Outport  Port=2
  wires:
  SSR4 to SSR8/1(Data Out) -> Multiport Switch/4
  SSR2 to SSR8/1(Data Out) -> Multiport Switch/3
  SSR1 to SSR8/1(Data Out) -> Multiport Switch/2
  Data In/1 -> SSR to Vector/1(SSR)
  Bit Slice1/1 -> SSR2 to SSR8/2(Index)
  HDL Counter/1 -> Bit Slice/1, Bit Slice1/1, SSR1 to SSR8/2(Index)
  SSR Control/1 -> Multiport Switch1/1, Multiport Switch/1
  Bit Slice/1 -> SSR4 to SSR8/2(Index)
  SSR1 to SSR8/2(Valid Out) -> Multiport Switch1/2
  SSR2 to SSR8/2(Valid Out) -> Multiport Switch1/3
  SSR4 to SSR8/2(Valid Out) -> Multiport Switch1/4
  Multiport Switch1/1 -> AND/1
  AND/1 -> Unit Delay Enabled Synchronous/2, Unit Delay/1
  Valid In/1 -> AND/2, Multiport Switch1/5, HDL Counter/1
  Unit Delay/1 -> Valid Out/1
  Multiport Switch/1 -> Unit Delay Enabled Synchronous/1
  Unit Delay Enabled Synchronous/1 -> Vector to SSR/1(Vector)
  SSR to Vector/1(Vector) -> Multiport Switch/5, SSR1 to SSR8/1(Data In), SSR2 to SSR8/1(Data In), SSR4 to SSR8/1(Data In)
  Vector to SSR/1(SSR) -> Data Out/1

== system mw_ssrconverter/Stimulus Imag/Vector to SSR ==
  Vector : Inport
  Bit Concat : hdlsllib/Logic and Bit Operations/Bit Concat  numInputs=8
  Selector0 : Selector  InputPortWidth=8  IndexOptions=Index vector (dialog)  Indices=8  OutputSizes=1
  Selector1 : Selector  InputPortWidth=8  IndexOptions=Index vector (dialog)  Indices=7  OutputSizes=1
  Selector2 : Selector  InputPortWidth=8  IndexOptions=Index vector (dialog)  Indices=6  OutputSizes=1
  Selector3 : Selector  InputPortWidth=8  IndexOptions=Index vector (dialog)  Indices=5  OutputSizes=1
  Selector4 : Selector  InputPortWidth=8  IndexOptions=Index vector (dialog)  Indices=4  OutputSizes=1
  Selector5 : Selector  InputPortWidth=8  IndexOptions=Index vector (dialog)  Indices=3  OutputSizes=1
  Selector6 : Selector  InputPortWidth=8  IndexOptions=Index vector (dialog)  Indices=2  OutputSizes=1
  Selector7 : Selector  InputPortWidth=8  IndexOptions=Index vector (dialog)  Indices=1  OutputSizes=1
  SSR : Outport
  wires:
  Selector7/1 -> Bit Concat/8
  Selector6/1 -> Bit Concat/7
  Selector5/1 -> Bit Concat/6
  Selector4/1 -> Bit Concat/5
  Selector3/1 -> Bit Concat/4
  Selector2/1 -> Bit Concat/3
  Selector1/1 -> Bit Concat/2
  Selector0/1 -> Bit Concat/1
  Vector/1 -> Selector0/1, Selector1/1, Selector2/1, Selector3/1, Selector4/1, Selector5/1, Selector7/1, Selector6/1
  Bit Concat/1 -> SSR/1

== system mw_ssrconverter/Stimulus Real/Vector to SSR ==
  Vector : Inport
  Bit Concat : hdlsllib/Logic and Bit Operations/Bit Concat  numInputs=8
  Selector0 : Selector  InputPortWidth=8  IndexOptions=Index vector (dialog)  Indices=8  OutputSizes=1
  Selector1 : Selector  InputPortWidth=8  IndexOptions=Index vector (dialog)  Indices=7  OutputSizes=1
  Selector2 : Selector  InputPortWidth=8  IndexOptions=Index vector (dialog)  Indices=6  OutputSizes=1
  Selector3 : Selector  InputPortWidth=8  IndexOptions=Index vector (dialog)  Indices=5  OutputSizes=1
  Selector4 : Selector  InputPortWidth=8  IndexOptions=Index vector (dialog)  Indices=4  OutputSizes=1
  Selector5 : Selector  InputPortWidth=8  IndexOptions=Index vector (dialog)  Indices=3  OutputSizes=1
  Selector6 : Selector  InputPortWidth=8  IndexOptions=Index vector (dialog)  Indices=2  OutputSizes=1
  Selector7 : Selector  InputPortWidth=8  IndexOptions=Index vector (dialog)  Indices=1  OutputSizes=1
  SSR : Outport
  wires:
  Bit Concat/1 -> SSR/1
  Vector/1 -> Selector6/1, Selector7/1, Selector5/1, Selector4/1, Selector3/1, Selector2/1, Selector1/1, Selector0/1
  Selector0/1 -> Bit Concat/1
  Selector1/1 -> Bit Concat/2
  Selector2/1 -> Bit Concat/3
  Selector3/1 -> Bit Concat/4
  Selector4/1 -> Bit Concat/5
  Selector5/1 -> Bit Concat/6
  Selector6/1 -> Bit Concat/7
  Selector7/1 -> Bit Concat/8

== system mw_ssrconverter/SSR Subset Converter/SSR Deserializer Imag/SSR to Vector ==
  SSR : Inport
  Bit Slice0 : hdlsllib/Logic and Bit Operations/Bit Slice  lidx=15  ridx=0
      settings: SourceProductBaseCode=SL
  Bit Slice1 : hdlsllib/Logic and Bit Operations/Bit Slice  lidx=31  ridx=16
      settings: SourceProductBaseCode=SL
  Bit Slice2 : hdlsllib/Logic and Bit Operations/Bit Slice  lidx=47  ridx=32
      settings: SourceProductBaseCode=SL
  Bit Slice3 : hdlsllib/Logic and Bit Operations/Bit Slice  lidx=63  ridx=48
      settings: SourceProductBaseCode=SL
  Bit Slice4 : hdlsllib/Logic and Bit Operations/Bit Slice  lidx=79  ridx=64
      settings: SourceProductBaseCode=SL
  Bit Slice5 : hdlsllib/Logic and Bit Operations/Bit Slice  lidx=95  ridx=80
      settings: SourceProductBaseCode=SL
  Bit Slice6 : hdlsllib/Logic and Bit Operations/Bit Slice  lidx=111  ridx=96
      settings: SourceProductBaseCode=SL
  Bit Slice7 : hdlsllib/Logic and Bit Operations/Bit Slice  lidx=127  ridx=112
      settings: SourceProductBaseCode=SL
  Matrix Concatenate : Concatenate  NumInputs=8  ConcatenateDimension=2
  Vector : Outport
  wires:
  Bit Slice7/1 -> Matrix Concatenate/8
  Bit Slice6/1 -> Matrix Concatenate/7
  Bit Slice5/1 -> Matrix Concatenate/6
  Bit Slice4/1 -> Matrix Concatenate/5
  Bit Slice3/1 -> Matrix Concatenate/4
  Bit Slice2/1 -> Matrix Concatenate/3
  Bit Slice1/1 -> Matrix Concatenate/2
  Bit Slice0/1 -> Matrix Concatenate/1
  SSR/1 -> Bit Slice0/1, Bit Slice1/1, Bit Slice2/1, Bit Slice3/1, Bit Slice4/1, Bit Slice5/1, Bit Slice7/1, Bit Slice6/1
  Matrix Concatenate/1 -> Vector/1

== system mw_ssrconverter/SSR Subset Converter/SSR Deserializer Imag/Subsystem ==
  Set : Inport
  Reset : Inport  Port=2
  Constant : Constant  OutDataTypeStr=boolean  SampleTime=-1
  Multiport Switch : MultiPortSwitch  DataPortOrder=Zero-based contiguous  Inputs=2  zeroidx=on
  Unit Delay Resettable Synchronous : hdlsllib/Discrete/Unit Delay Resettable Synchronous  InitialCondition=0.0  SampleTime=-1
      settings: SourceProductBaseCode=SL
  Latch : Outport
  wires:
  Multiport Switch/1 -> Unit Delay Resettable Synchronous/1, Latch/1
  Set/1 -> Multiport Switch/1
  Reset/1 -> Unit Delay Resettable Synchronous/2
  Constant/1 -> Multiport Switch/3
  Unit Delay Resettable Synchronous/1 -> Multiport Switch/2

== system mw_ssrconverter/SSR Subset Converter/SSR Deserializer Imag/Subsystem1 ==
  Set : Inport
  Reset : Inport  Port=2
  Constant : Constant  OutDataTypeStr=boolean  SampleTime=-1
  Multiport Switch : MultiPortSwitch  DataPortOrder=Zero-based contiguous  Inputs=2  zeroidx=on
  Unit Delay Resettable Synchronous : hdlsllib/Discrete/Unit Delay Resettable Synchronous  InitialCondition=0.0  SampleTime=-1
      settings: SourceProductBaseCode=SL
  Latch : Outport
  wires:
  Unit Delay Resettable Synchronous/1 -> Multiport Switch/2
  Constant/1 -> Multiport Switch/3
  Reset/1 -> Unit Delay Resettable Synchronous/2
  Set/1 -> Multiport Switch/1
  Multiport Switch/1 -> Latch/1, Unit Delay Resettable Synchronous/1

== system mw_ssrconverter/SSR Subset Converter/SSR Deserializer Real/SSR to Vector ==
  SSR : Inport
  Bit Slice0 : hdlsllib/Logic and Bit Operations/Bit Slice  lidx=15  ridx=0
      settings: SourceProductBaseCode=SL
  Bit Slice1 : hdlsllib/Logic and Bit Operations/Bit Slice  lidx=31  ridx=16
      settings: SourceProductBaseCode=SL
  Bit Slice2 : hdlsllib/Logic and Bit Operations/Bit Slice  lidx=47  ridx=32
      settings: SourceProductBaseCode=SL
  Bit Slice3 : hdlsllib/Logic and Bit Operations/Bit Slice  lidx=63  ridx=48
      settings: SourceProductBaseCode=SL
  Bit Slice4 : hdlsllib/Logic and Bit Operations/Bit Slice  lidx=79  ridx=64
      settings: SourceProductBaseCode=SL
  Bit Slice5 : hdlsllib/Logic and Bit Operations/Bit Slice  lidx=95  ridx=80
      settings: SourceProductBaseCode=SL
  Bit Slice6 : hdlsllib/Logic and Bit Operations/Bit Slice  lidx=111  ridx=96
      settings: SourceProductBaseCode=SL
  Bit Slice7 : hdlsllib/Logic and Bit Operations/Bit Slice  lidx=127  ridx=112
      settings: SourceProductBaseCode=SL
  Matrix Concatenate : Concatenate  NumInputs=8  ConcatenateDimension=2
  Vector : Outport
  wires:
  Matrix Concatenate/1 -> Vector/1
  SSR/1 -> Bit Slice6/1, Bit Slice7/1, Bit Slice5/1, Bit Slice4/1, Bit Slice3/1, Bit Slice2/1, Bit Slice1/1, Bit Slice0/1
  Bit Slice0/1 -> Matrix Concatenate/1
  Bit Slice1/1 -> Matrix Concatenate/2
  Bit Slice2/1 -> Matrix Concatenate/3
  Bit Slice3/1 -> Matrix Concatenate/4
  Bit Slice4/1 -> Matrix Concatenate/5
  Bit Slice5/1 -> Matrix Concatenate/6
  Bit Slice6/1 -> Matrix Concatenate/7
  Bit Slice7/1 -> Matrix Concatenate/8

== system mw_ssrconverter/SSR Subset Converter/SSR Deserializer Real/Subsystem ==
  Set : Inport
  Reset : Inport  Port=2
  Constant : Constant  OutDataTypeStr=boolean  SampleTime=-1
  Multiport Switch : MultiPortSwitch  DataPortOrder=Zero-based contiguous  Inputs=2  zeroidx=on
  Unit Delay Resettable Synchronous : hdlsllib/Discrete/Unit Delay Resettable Synchronous  InitialCondition=0.0  SampleTime=-1
      settings: SourceProductBaseCode=SL
  Latch : Outport
  wires:
  Unit Delay Resettable Synchronous/1 -> Multiport Switch/2
  Constant/1 -> Multiport Switch/3
  Reset/1 -> Unit Delay Resettable Synchronous/2
  Set/1 -> Multiport Switch/1
  Multiport Switch/1 -> Latch/1, Unit Delay Resettable Synchronous/1

== system mw_ssrconverter/SSR Subset Converter/SSR Deserializer Real/Subsystem1 ==
  Set : Inport
  Reset : Inport  Port=2
  Constant : Constant  OutDataTypeStr=boolean  SampleTime=-1
  Multiport Switch : MultiPortSwitch  DataPortOrder=Zero-based contiguous  Inputs=2  zeroidx=on
  Unit Delay Resettable Synchronous : hdlsllib/Discrete/Unit Delay Resettable Synchronous  InitialCondition=0.0  SampleTime=-1
      settings: SourceProductBaseCode=SL
  Latch : Outport
  wires:
  Multiport Switch/1 -> Unit Delay Resettable Synchronous/1, Latch/1
  Set/1 -> Multiport Switch/1
  Reset/1 -> Unit Delay Resettable Synchronous/2
  Constant/1 -> Multiport Switch/3
  Unit Delay Resettable Synchronous/1 -> Multiport Switch/2
